simulink model "Traffic_Light"  (R2022b)
settings: Solver=VariableStepAuto  StartTime=0.0  StopTime=31  RelTol=1e-3
settings Model: Creator=davit  LastModifiedBy=Soumya Ranjan
settings SolverCC: AlgebraicLoopSolver=TrustRegion
settings DataIOCC: ReturnWorkspaceOutputs=off
settings DebuggingCC: UnconnectedInputMsg=warning  UnconnectedOutputMsg=warning  UnconnectedLineMsg=warning  SFMachineParentedDataDiag=warning  ArithmeticOperatorsInVariantConditions=warning
settings ModelReferenceCC: EnableRefExpFcnMdlSchedulingChecks=on
settings SFSimCC: SimUseLocalCustomCode=off  CustomCodeUndefinedFunction=UseInterfaceOnly
settings RTWCC: RTWUseLocalCustomCode=off

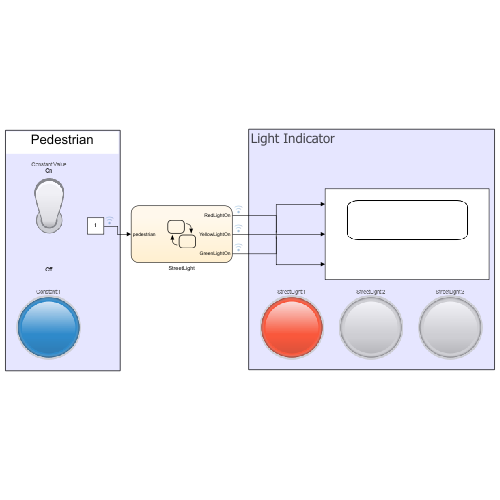
[thumbnail: Simulink's stored preview of the top-level diagram]
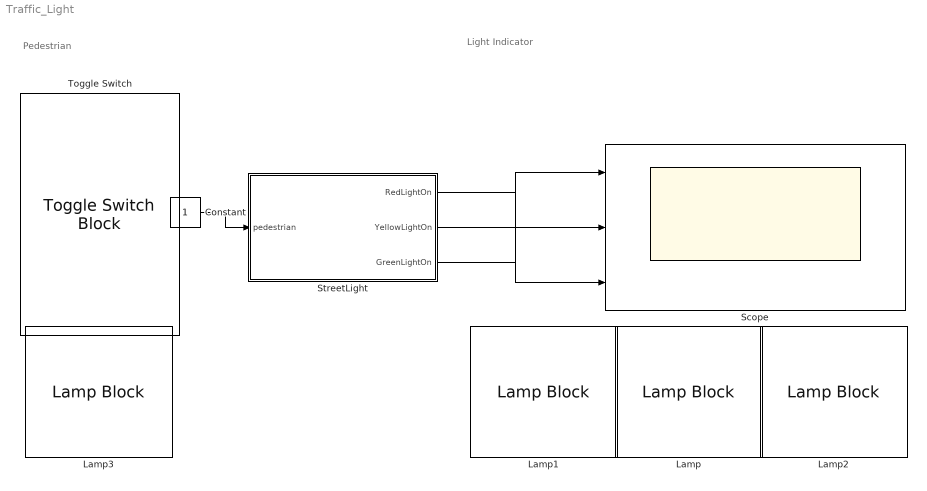
== system Traffic_Light ==
  note: Pedestrian
  note: Light Indicator
  Constant : Constant  OutDataTypeStr=boolean
  Lamp{,1..3} (4 alike) : LampBlock
  Scope : Scope  NumInputPorts=3
  StreetLight : Stateflow chart  TreatAsAtomicUnit=on
  Toggle Switch : ToggleSwitchBlock
      settings: Values={{'Off', 'On'}, [0 1]}
  wires:
  Constant/1 -> StreetLight/1(pedestrian)
  StreetLight/1(RedLightOn) -> Scope/3
  StreetLight/3(GreenLightOn) -> Scope/1
  StreetLight/2(YellowLightOn) -> Scope/2

== stateflow chart Traffic_Light/StreetLight ==
  state GreenLightOn
    entry:
    RedLightOn=0;
    GreenLightOn=1;
    YellowLightOn=0;
  state RedLightOn
    entry:
    RedLightOn=1;
    GreenLightOn=0;
    YellowLightOn=0;
  state pedestrian
  state YellowLightOn
    entry:
    RedLightOn=0;
    GreenLightOn=0;
    YellowLightOn=1;
  (default) -> RedLightOn
  RedLightOn -> GreenLightOn : after(10,sec){GreenLightOn}
  pedestrian -> GreenLightOn
  GreenLightOn -> YellowLightOn [order 2] : after(20,sec)[pedestrian==1]{YellowLightOn}
  GreenLightOn -> YellowLightOn [order 1] : after(10,sec)[pedestrian==0]{YellowLightOn}
  YellowLightOn -> RedLightOn : after(3,sec){RedLightOn}
  data: RedLightOn output; pedestrian input boolean =false; YellowLightOn output; GreenLightOn output
